simulink model "PV"  (R2024a)
settings: Solver=VariableStepAuto  StartTime=0.0  StopTime=0.5  RelTol=1e-3
libraries: ee_lib x48, nesl_utility x5, fl_lib x4, simulink x1, spspowerguiLib x1
settings Model: Creator=hp  LastModifiedBy=hp

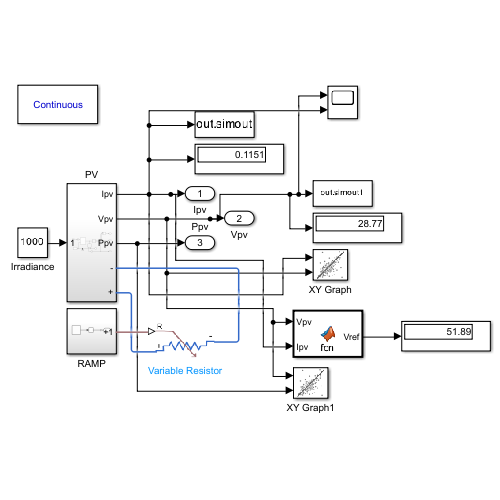
[thumbnail: Simulink's stored preview of the top-level diagram]
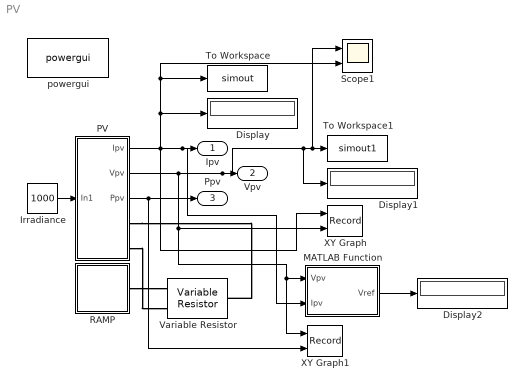
== system PV ==
  Display : Display
  Display1 : Display
  Display2 : Display
  Irradiance : Constant  Value=1000
  MATLAB Function : MATLAB Function  TreatAsAtomicUnit=on
  PV : Subsystem
  RAMP : Subsystem
  Scope1 : Scope  NumInputPorts=2
  To Workspace : ToWorkspace  VariableName=simout  SaveFormat=Timeseries  SampleTime=-1
  To Workspace1 : ToWorkspace  VariableName=simout1  SaveFormat=Timeseries  SampleTime=-1
  Variable Resistor : fl_lib/Electrical/Electrical Elements/Variable Resistor  Rmin=0 Ohm  thermalEnable=false  thermal_mass=1 J/K  i_specify=off  i_priority=None  i=0 A  i_nominal_specify=off  i_nominal_value=1  i_nominal_unit=A  v_specify=off  v_priority=None  v=0 V  v_nominal_specify=off  v_nominal_value=1  v_nominal_unit=V  T_specify=off  T_priority=None  T=300 K  T_nominal_specify=off  T_nominal_value=1  T_nominal_unit=K
  XY Graph : Record  FileSettingsInternal="{\"entries\":[{\"content\":{\"excelSettings\":{\"content\":{},\"type\":\"Streamout.ExcelSettings\"}},\"type\":\"Streamout.FileSettingStorage\",\"uuid\":\"\"}],\"packageUris\":[\"http:\\/\\/schema.mathworks.com\\/mf0\\/streamout_blocks\\/R2020a\"],\"version\":\"1.0\"}"  Layout=[1 1]  SignalsInternal="{\"entries\":[{\"content\":{\"signals\":[{\"content\":{\"blockPath\":[],\"dimensions\":[1],\"domain\":\"\",\"lineColor\":\"#a2142f\",\"plots\":[ 1 ],\"port\":1,\"signalID\":1,\"signalName\":\"PV:1\"},\"type\":\"RecordBlkView.Signal\",\"uuid\":\"\"},{\"content\":{\"blockPath\":[],\"dimensions\":[1],\"domain\":\"\",\"lineColor\":\"#139fff\",\"plots\":[ 1 ],\"port\":2,\"signalID\":2,\"signalName\":\"PV:2\"},\"type\":\"RecordBlkView.Signal\",\"uuid\":\"\"}]},\"type\":\"RecordBlkView.InputSignals\",\"uuid\":\"\"}],\"packageUris\":[\"http:\\/\\/schema.mathworks.com\\/mf0\\/streamout_blocks\\/R2020a\"],\"version\":\"1.0\"}"  VisualizationBindings="{\"xyplotplugin\":{\"info\":[{\"series\":[{\"bindingParametersList\":[{\"parameter\":\"X-Axis\",\"signalID\":1,\"signalName\":\"PV:1\"},{\"parameter\":\"Y-Axis\",\"signalID\":2,\"signalName\":\"PV:2\"}],\"seriesID\":0}],\"subplotID\":1}]}}"  CompatibilityTag=XY
  XY Graph1 : Record  FileSettingsInternal="{\"entries\":[{\"content\":{\"excelSettings\":{\"content\":{},\"type\":\"Streamout.ExcelSettings\"}},\"type\":\"Streamout.FileSettingStorage\",\"uuid\":\"\"}],\"packageUris\":[\"http:\\/\\/schema.mathworks.com\\/mf0\\/streamout_blocks\\/R2020a\"],\"version\":\"1.0\"}"  Layout=[1 1]  SignalsInternal="{\"entries\":[{\"content\":{\"signals\":[{\"content\":{\"blockPath\":[],\"dimensions\":[1],\"domain\":\"\",\"lineColor\":\"#a2142f\",\"plots\":[ 1 ],\"port\":1,\"signalID\":1,\"signalName\":\"Vpv\"},\"type\":\"RecordBlkView.Signal\",\"uuid\":\"\"},{\"content\":{\"blockPath\":[],\"dimensions\":[1],\"domain\":\"\",\"lineColor\":\"#139fff\",\"plots\":[ 1 ],\"port\":2,\"signalID\":2,\"signalName\":\"Ppv\"},\"type\":\"RecordBlkView.Signal\",\"uuid\":\"\"}]},\"type\":\"RecordBlkView.InputSignals\",\"uuid\":\"\"}],\"packageUris\":[\"http:\\/\\/schema.mathworks.com\\/mf0\\/streamout_blocks\\/R2020a\"],\"version\":\"1.0\"}"  VisualizationBindings="{\"xyplotplugin\":{\"info\":[{\"series\":[{\"bindingParametersList\":[{\"parameter\":\"X-Axis\",\"signalID\":1,\"signalName\":\"Vpv\"},{\"parameter\":\"Y-Axis\",\"signalID\":2,\"signalName\":\"Ppv\"}],\"seriesID\":0}],\"subplotID\":1}]}}"  CompatibilityTag=XY
  powergui : spspowerguiLib/powergui  Priority=1  SimulationMode=Continuous  SampleTime=50e-6  frequency=60  Iterations=50  frequencyindice=60  Pbase=100e6  ErrMax=1e-4  UnitsV=kV  UnitsW=MW  buscounter=0  FunctionMessages=off  echomessages=off  EnableUseOfTLC=off  CurrentSourceSwitches=off  DisableSnubberDevices=off  DisableRonSwitches=off  DisableVfSwitches=off  DisplayEquations=off  AutomaticDiscreteSolvers=off  SolverType=Tustin/Backward Euler (TBE)  Interpol=off  ExternalGateDelay=off  methode=off  Ts=100  x0status=blocks  SPID=on  SwTol=0  HookPort=off  NonlinearTolerance=1e-4  nMaxIteration=100  ContinueOnMaxIteration=off  RestoreLinks=warning  ResistiveCurrentMeasurement=off  Frange=[0:2:500]  Ylog=off  Xlog=on  ShowGrid=off  save=off  variable=ZData  structure=0  ZoomFFT=off  StartTime=0.0  cycles=1  DisplayStyle=1  fundamental=60  FreqAxis=off  MaxFrequency=1000  frequencyindicesteady=1  RmsSteady=1  display=off
  Ipv : Outport
  Vpv : Outport  Port=2
  Ppv : Outport  Port=3
  wires:
  Irradiance/1 -> PV/1(In1)
  PV/1(Ipv) -> XY Graph/1, Scope1/2, To Workspace/1, Display/1, MATLAB Function/2(Ipv), Ipv/1
  PV/3(Ppv) -> XY Graph1/2, Ppv/1
  PV/2(Vpv) -> XY Graph1/1, MATLAB Function/1(Vpv), XY Graph/2, Vpv/1, Scope1/1, To Workspace1/1, Display1/1
  MATLAB Function/1(Vref) -> Display2/1
  connections:
  PV/RConn2 -- Variable Resistor/LConn2
  PV/RConn1 -- Variable Resistor/RConn1
  RAMP/RConn1 -- Variable Resistor/LConn1

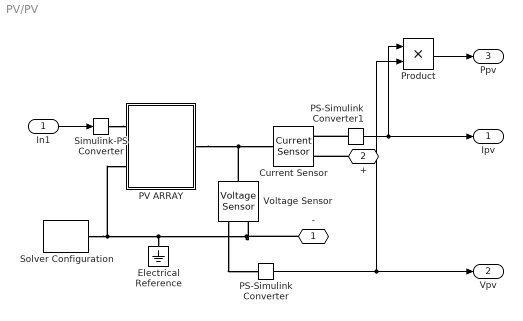
== system PV/PV ==
  In1 : Inport
  Current Sensor : fl_lib/Electrical/Electrical Sensors/Current Sensor
  Electrical Reference : fl_lib/Electrical/Electrical Elements/Electrical Reference
  PS-Simulink Converter : nesl_utility/PS-Simulink Converter  PhysicalDomain=network_engine_domain  SubClassName=ps_output  LeftPortType=input  RightPortType=output  PseudoPeriodic=off  Frequencies=[]  VectorFormat=inherit  Unit=inherit  AffineConversion=off
  PS-Simulink Converter1 : nesl_utility/PS-Simulink Converter  PhysicalDomain=network_engine_domain  SubClassName=ps_output  LeftPortType=input  RightPortType=output  PseudoPeriodic=off  Frequencies=[]  VectorFormat=inherit  Unit=inherit  AffineConversion=off
  PV ARRAY : Subsystem
  Product : Product
  Simulink-PS Converter : nesl_utility/Simulink-PS Converter  PhysicalDomain=network_engine_domain  SubClassName=ps_input  LeftPortType=input  RightPortType=output  PseudoPeriodic=off  Frequencies=[]  NoiseDistribution=none  NoiseParameters=[]  Unit=1  AffineConversion=off  FilteringAndDerivatives=provide  SimscapeFilterOrder=1  InputFilterTimeConstant=0.001  UdotUserProvided=0
  Solver Configuration : nesl_utility/Solver Configuration  PhysicalDomain=network_engine_domain  SubClassName=solver  LeftPortType=input  RightPortType=generic  Tones=[]  Harmonics=[]  SimulateNoise=off  Profile=off  UseLocalSampling=off  EnableSwitchedLinearOptims=on  FrequencyDomain=off  UseCCode=off  RelTol=0.001  AbsTol=0.001  MinStep=1e-09  ToWorkspace=off  RevertToSquareIcSolve=off  NumHomotopyIterations=100  PhasorMode=off  PhasorModeNumHarmonics=1  ConsistencySolver=NEWTON_XTOL_AFTER_FTOL  IndexReductionMethod=DerivativeReplacement  DoDC=off  ResidualTolerance=1e-09  ConsistencyTolSource=GLOBAL  ConsistencyAbsTol=0.001  ConsistencyRelTol=0.001  ConsistencyTolFactor=0.001  UseLocalSolver=off  LocalSolverChoice=NE_BACKWARD_EULER_ADVANCER  ResolveIndetEquations=on  FunctionEvalNumThread=1  LocalSolverSampleTime=0.001  DoFixedCost=off  MaxNonlinIter=3  MaxModeIter=2  ComputeImpulses=off  ImpulseIterations=2  LinearAlgebra=auto  LinearAlgebraNumThread=0  EquationFormulation=NE_TIME_EF  DelaysMemoryBudget=1024  AutomaticFiltering=on  FilteringTimeConstant=0.001  PartitionStorageMethod=AS_NEEDED  PartitionMemoryBudget=1024  PartitionMethod=ROBUST  MultibodyUseLocalSolver=off  MultibodyLocalSolverChoice=ODE1  MultibodyLocalSolverSampleTime=0.001
  Voltage Sensor : fl_lib/Electrical/Electrical Sensors/Voltage Sensor
  - : PMIOPort  Side=Right
  + : PMIOPort  Port=2  Side=Right
  Ipv : Outport
  Vpv : Outport  Port=2
  Ppv : Outport  Port=3
  wires:
  PS-Simulink Converter1/1 -> Ipv/1, Product/1
  PS-Simulink Converter/1 -> Vpv/1, Product/2
  Product/1 -> Ppv/1
  In1/1 -> Simulink-PS Converter/1
  connections:
  PS-Simulink Converter1/LConn1 -- Current Sensor/RConn1
  Simulink-PS Converter/RConn1 -- PV ARRAY/LConn1
  +/RConn1 -- Current Sensor/RConn2
  PV ARRAY/RConn1 -- Voltage Sensor/LConn1 -- Current Sensor/LConn1
  Solver Configuration/RConn1 -- -/RConn1 -- Voltage Sensor/RConn2 -- Electrical Reference/LConn1 -- PV ARRAY/LConn2
  Voltage Sensor/RConn1 -- PS-Simulink Converter/LConn1

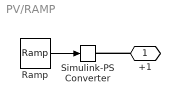
== system PV/RAMP ==
  Ramp : simulink/Sources/Ramp  slope=500  start=0  InitialOutput=0
  Simulink-PS Converter : nesl_utility/Simulink-PS Converter  PhysicalDomain=network_engine_domain  SubClassName=ps_input  LeftPortType=input  RightPortType=output  PseudoPeriodic=off  Frequencies=[]  NoiseDistribution=none  NoiseParameters=[]  Unit=1  AffineConversion=off  FilteringAndDerivatives=provide  SimscapeFilterOrder=1  InputFilterTimeConstant=0.001  UdotUserProvided=0
  +1 : PMIOPort  Side=Right
  wires:
  Ramp/1 -> Simulink-PS Converter/1
  connections:
  +1/RConn1 -- Simulink-PS Converter/RConn1

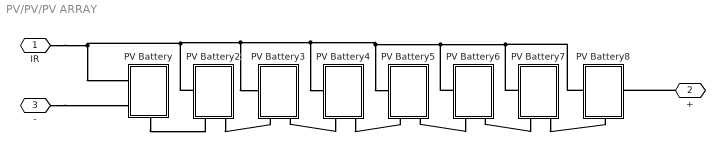
== system PV/PV/PV ARRAY ==
  PV Battery : Subsystem
      settings: PortSchema="{\"entries\":[{\"content\":{\"sides\":[{\"content\":{\"connectorIds\":[\"LConn1\",\"LConn2\"]},\"type\":\"ConnectorPlacement.EquallySpacedRectSide\",\"uuid\":\"343a5c80-c490-4c63-968f-4227f8b0bc69\"},{\"content\":{\"side\":\"RIGHT\"},\"type\":\"ConnectorPlacement.EquallySpacedRectSide\",\"uuid\":\"ee4aa178-7663-40d5-bcc3-f91d4c44b2a7\"},{\"content\":{\"side\":\"TOP\"},\"type\":\"ConnectorPlacement.EquallySpacedRectSide\",\"uuid\":\"a03aa1aa-4889-4cfe-9c8f-92adc9f70735\"},{\"content\":{\"connectorIds\":[\"RConn1\"],\"side\":\"BOTTOM\"},\"type\":\"ConnectorPlacement.EquallySpacedRectSide\",\"uuid\":\"9e292261-11b5-43da-a6bc-bd19848d4a2b\"}]},\"type\":\"ConnectorPlacement.EquallySpacedConnector\",\"uuid\":\"be6337a3-66bb-48d6-bc68-5a7e39297b74\"}],\"packageUris\":[\"http://schema.mathworks.com/mf0/Connector/R2020b\"],\"version\":\"1.0\"}"
  PV Battery2 : Subsystem
      settings: PortSchema="{\"entries\":[{\"content\":{\"sides\":[{\"content\":{\"connectorIds\":[\"LConn1\"]},\"type\":\"ConnectorPlacement.EquallySpacedRectSide\",\"uuid\":\"343a5c80-c490-4c63-968f-4227f8b0bc69\"},{\"content\":{\"side\":\"RIGHT\"},\"type\":\"ConnectorPlacement.EquallySpacedRectSide\",\"uuid\":\"ee4aa178-7663-40d5-bcc3-f91d4c44b2a7\"},{\"content\":{\"side\":\"TOP\"},\"type\":\"ConnectorPlacement.EquallySpacedRectSide\",\"uuid\":\"a03aa1aa-4889-4cfe-9c8f-92adc9f70735\"},{\"content\":{\"connectorIds\":[\"RConn1\",\"RConn2\"],\"side\":\"BOTTOM\"},\"type\":\"ConnectorPlacement.EquallySpacedRectSide\",\"uuid\":\"35521834-7b12-4f19-8790-069a58e4d08c\"}]},\"type\":\"ConnectorPlacement.EquallySpacedConnector\",\"uuid\":\"be6337a3-66bb-48d6-bc68-5a7e39297b74\"}],\"packageUris\":[\"http://schema.mathworks.com/mf0/Connector/R2020b\"],\"version\":\"1.0\"}"
  PV Battery3 : Subsystem
      settings: PortSchema="{\"entries\":[{\"content\":{\"sides\":[{\"content\":{\"connectorIds\":[\"LConn1\"]},\"type\":\"ConnectorPlacement.EquallySpacedRectSide\",\"uuid\":\"343a5c80-c490-4c63-968f-4227f8b0bc69\"},{\"content\":{\"side\":\"RIGHT\"},\"type\":\"ConnectorPlacement.EquallySpacedRectSide\",\"uuid\":\"ee4aa178-7663-40d5-bcc3-f91d4c44b2a7\"},{\"content\":{\"side\":\"TOP\"},\"type\":\"ConnectorPlacement.EquallySpacedRectSide\",\"uuid\":\"a03aa1aa-4889-4cfe-9c8f-92adc9f70735\"},{\"content\":{\"connectorIds\":[\"RConn1\",\"RConn2\"],\"side\":\"BOTTOM\"},\"type\":\"ConnectorPlacement.EquallySpacedRectSide\",\"uuid\":\"3f39185d-c5ea-40de-b77a-797dfb5d777b\"}]},\"type\":\"ConnectorPlacement.EquallySpacedConnector\",\"uuid\":\"be6337a3-66bb-48d6-bc68-5a7e39297b74\"}],\"packageUris\":[\"http://schema.mathworks.com/mf0/Connector/R2020b\"],\"version\":\"1.0\"}"
  PV Battery4 : Subsystem
      settings: PortSchema="{\"entries\":[{\"content\":{\"sides\":[{\"content\":{\"connectorIds\":[\"LConn1\"]},\"type\":\"ConnectorPlacement.EquallySpacedRectSide\",\"uuid\":\"343a5c80-c490-4c63-968f-4227f8b0bc69\"},{\"content\":{\"side\":\"RIGHT\"},\"type\":\"ConnectorPlacement.EquallySpacedRectSide\",\"uuid\":\"ee4aa178-7663-40d5-bcc3-f91d4c44b2a7\"},{\"content\":{\"side\":\"TOP\"},\"type\":\"ConnectorPlacement.EquallySpacedRectSide\",\"uuid\":\"a03aa1aa-4889-4cfe-9c8f-92adc9f70735\"},{\"content\":{\"connectorIds\":[\"RConn1\",\"RConn2\"],\"side\":\"BOTTOM\"},\"type\":\"ConnectorPlacement.EquallySpacedRectSide\",\"uuid\":\"6de3b158-1ff0-4b44-8b1b-28764e596168\"}]},\"type\":\"ConnectorPlacement.EquallySpacedConnector\",\"uuid\":\"be6337a3-66bb-48d6-bc68-5a7e39297b74\"}],\"packageUris\":[\"http://schema.mathworks.com/mf0/Connector/R2020b\"],\"version\":\"1.0\"}"
  PV Battery5 : Subsystem
      settings: PortSchema="{\"entries\":[{\"content\":{\"sides\":[{\"content\":{\"connectorIds\":[\"LConn1\"]},\"type\":\"ConnectorPlacement.EquallySpacedRectSide\",\"uuid\":\"343a5c80-c490-4c63-968f-4227f8b0bc69\"},{\"content\":{\"side\":\"RIGHT\"},\"type\":\"ConnectorPlacement.EquallySpacedRectSide\",\"uuid\":\"ee4aa178-7663-40d5-bcc3-f91d4c44b2a7\"},{\"content\":{\"side\":\"TOP\"},\"type\":\"ConnectorPlacement.EquallySpacedRectSide\",\"uuid\":\"a03aa1aa-4889-4cfe-9c8f-92adc9f70735\"},{\"content\":{\"connectorIds\":[\"RConn1\",\"RConn2\"],\"side\":\"BOTTOM\"},\"type\":\"ConnectorPlacement.EquallySpacedRectSide\",\"uuid\":\"8bb7a49a-a7b0-4dc7-aec8-a84a106abde2\"}]},\"type\":\"ConnectorPlacement.EquallySpacedConnector\",\"uuid\":\"be6337a3-66bb-48d6-bc68-5a7e39297b74\"}],\"packageUris\":[\"http://schema.mathworks.com/mf0/Connector/R2020b\"],\"version\":\"1.0\"}"
  PV Battery6 : Subsystem
      settings: PortSchema="{\"entries\":[{\"content\":{\"sides\":[{\"content\":{\"connectorIds\":[\"LConn1\"]},\"type\":\"ConnectorPlacement.EquallySpacedRectSide\",\"uuid\":\"343a5c80-c490-4c63-968f-4227f8b0bc69\"},{\"content\":{\"side\":\"RIGHT\"},\"type\":\"ConnectorPlacement.EquallySpacedRectSide\",\"uuid\":\"ee4aa178-7663-40d5-bcc3-f91d4c44b2a7\"},{\"content\":{\"side\":\"TOP\"},\"type\":\"ConnectorPlacement.EquallySpacedRectSide\",\"uuid\":\"a03aa1aa-4889-4cfe-9c8f-92adc9f70735\"},{\"content\":{\"connectorIds\":[\"RConn1\",\"RConn2\"],\"side\":\"BOTTOM\"},\"type\":\"ConnectorPlacement.EquallySpacedRectSide\",\"uuid\":\"8bb7a49a-a7b0-4dc7-aec8-a84a106abde2\"}]},\"type\":\"ConnectorPlacement.EquallySpacedConnector\",\"uuid\":\"be6337a3-66bb-48d6-bc68-5a7e39297b74\"}],\"packageUris\":[\"http://schema.mathworks.com/mf0/Connector/R2020b\"],\"version\":\"1.0\"}"
  PV Battery7 : Subsystem
      settings: PortSchema="{\"entries\":[{\"content\":{\"sides\":[{\"content\":{\"connectorIds\":[\"LConn1\"]},\"type\":\"ConnectorPlacement.EquallySpacedRectSide\",\"uuid\":\"343a5c80-c490-4c63-968f-4227f8b0bc69\"},{\"content\":{\"side\":\"RIGHT\"},\"type\":\"ConnectorPlacement.EquallySpacedRectSide\",\"uuid\":\"ee4aa178-7663-40d5-bcc3-f91d4c44b2a7\"},{\"content\":{\"side\":\"TOP\"},\"type\":\"ConnectorPlacement.EquallySpacedRectSide\",\"uuid\":\"a03aa1aa-4889-4cfe-9c8f-92adc9f70735\"},{\"content\":{\"connectorIds\":[\"RConn1\",\"RConn2\"],\"side\":\"BOTTOM\"},\"type\":\"ConnectorPlacement.EquallySpacedRectSide\",\"uuid\":\"8bb7a49a-a7b0-4dc7-aec8-a84a106abde2\"}]},\"type\":\"ConnectorPlacement.EquallySpacedConnector\",\"uuid\":\"be6337a3-66bb-48d6-bc68-5a7e39297b74\"}],\"packageUris\":[\"http://schema.mathworks.com/mf0/Connector/R2020b\"],\"version\":\"1.0\"}"
  PV Battery8 : Subsystem
      settings: PortSchema="{\"entries\":[{\"content\":{\"sides\":[{\"content\":{\"connectorIds\":[\"LConn1\"]},\"type\":\"ConnectorPlacement.EquallySpacedRectSide\",\"uuid\":\"343a5c80-c490-4c63-968f-4227f8b0bc69\"},{\"content\":{\"connectorIds\":[\"RConn1\"],\"side\":\"RIGHT\"},\"type\":\"ConnectorPlacement.EquallySpacedRectSide\",\"uuid\":\"ee4aa178-7663-40d5-bcc3-f91d4c44b2a7\"},{\"content\":{\"side\":\"TOP\"},\"type\":\"ConnectorPlacement.EquallySpacedRectSide\",\"uuid\":\"a03aa1aa-4889-4cfe-9c8f-92adc9f70735\"},{\"content\":{\"connectorIds\":[\"RConn2\"],\"side\":\"BOTTOM\"},\"type\":\"ConnectorPlacement.EquallySpacedRectSide\",\"uuid\":\"8bb7a49a-a7b0-4dc7-aec8-a84a106abde2\"}]},\"type\":\"ConnectorPlacement.EquallySpacedConnector\",\"uuid\":\"be6337a3-66bb-48d6-bc68-5a7e39297b74\"}],\"packageUris\":[\"http://schema.mathworks.com/mf0/Connector/R2020b\"],\"version\":\"1.0\"}"
  IR : PMIOPort  Side=Left
  + : PMIOPort  Port=2  Side=Right
  - : PMIOPort  Port=3  Side=Left
  connections:
  PV Battery2/LConn1 -- IR/RConn1 -- PV Battery/LConn1 -- PV Battery6/LConn1 -- PV Battery8/LConn1 -- PV Battery7/LConn1 -- PV Battery5/LConn1 -- PV Battery4/LConn1 -- PV Battery3/LConn1
  PV Battery/RConn1 -- PV Battery2/RConn1
  -/RConn1 -- PV Battery/LConn2
  PV Battery7/RConn2 -- PV Battery8/RConn2
  PV Battery2/RConn2 -- PV Battery3/RConn1
  PV Battery6/RConn1 -- PV Battery5/RConn2
  PV Battery4/RConn1 -- PV Battery3/RConn2
  PV Battery4/RConn2 -- PV Battery5/RConn1
  +/RConn1 -- PV Battery8/RConn1
  PV Battery7/RConn1 -- PV Battery6/RConn2

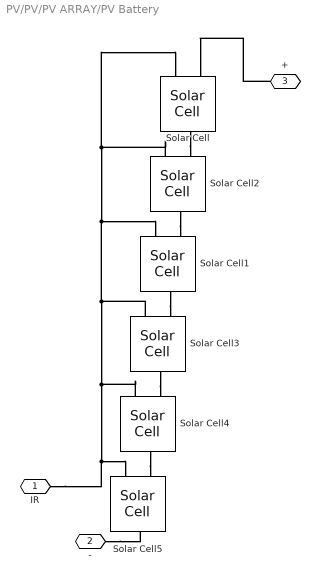
== system PV/PV/PV ARRAY/PV Battery ==
  Solar Cell{,1..5} (6 alike) : ee_lib/Sources/Solar Cell  prm=1  Isc=7.34 A  Voc=0.6 V  Is=1e-6 A  Is2=0 A  Iph=7.34 A  Ir0=1000 W/m^2  ec=1.5  N2=2  Rs=0 Ohm  Rp=inf Ohm  N_series=1  N_parallel=1  TIPH1=0 1/K  EG=1.11 eV  TXIS1=3  TXIS2=3  TRS1=0  TRP1=0  Tmeas=25 degC  TFIXED=25 degC  thermal_mass=100 J/K  initial_temperature=25 degC
  IR : PMIOPort  Side=Left
  - : PMIOPort  Port=2  Side=Left
  + : PMIOPort  Port=3  Side=Right
  connections:
  Solar Cell2/LConn1 -- Solar Cell/LConn1 -- Solar Cell3/LConn1 -- Solar Cell4/LConn1 -- IR/RConn1 -- Solar Cell5/LConn1 -- Solar Cell1/LConn1
  Solar Cell/RConn1 -- Solar Cell2/LConn2
  Solar Cell4/RConn1 -- Solar Cell5/LConn2
  +/RConn1 -- Solar Cell/LConn2
  Solar Cell1/RConn1 -- Solar Cell3/LConn2
  Solar Cell3/RConn1 -- Solar Cell4/LConn2
  -/RConn1 -- Solar Cell5/RConn1
  Solar Cell2/RConn1 -- Solar Cell1/LConn2

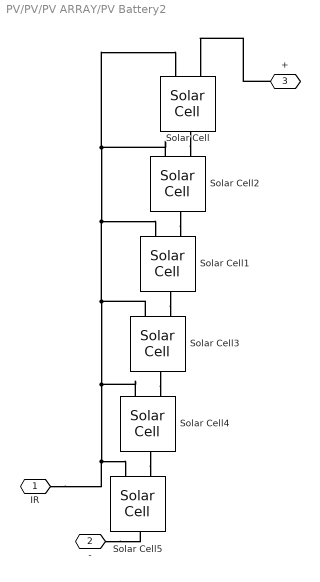
== system PV/PV/PV ARRAY/PV Battery2 ==
  Solar Cell{,1..5} (6 alike) : ee_lib/Sources/Solar Cell  prm=1  Isc=7.34 A  Voc=0.6 V  Is=1e-6 A  Is2=0 A  Iph=7.34 A  Ir0=1000 W/m^2  ec=1.5  N2=2  Rs=0 Ohm  Rp=inf Ohm  N_series=1  N_parallel=1  TIPH1=0 1/K  EG=1.11 eV  TXIS1=3  TXIS2=3  TRS1=0  TRP1=0  Tmeas=25 degC  TFIXED=25 degC  thermal_mass=100 J/K  initial_temperature=25 degC
  IR : PMIOPort  Side=Left
  - : PMIOPort  Port=2  Side=Right
  + : PMIOPort  Port=3  Side=Right
  connections:
  Solar Cell4/LConn1 -- Solar Cell3/LConn1 -- Solar Cell2/LConn1 -- Solar Cell/LConn1 -- Solar Cell1/LConn1 -- Solar Cell5/LConn1 -- IR/RConn1
  Solar Cell/RConn1 -- Solar Cell2/LConn2
  Solar Cell4/RConn1 -- Solar Cell5/LConn2
  +/RConn1 -- Solar Cell/LConn2
  Solar Cell1/RConn1 -- Solar Cell3/LConn2
  Solar Cell3/RConn1 -- Solar Cell4/LConn2
  -/RConn1 -- Solar Cell5/RConn1
  Solar Cell2/RConn1 -- Solar Cell1/LConn2

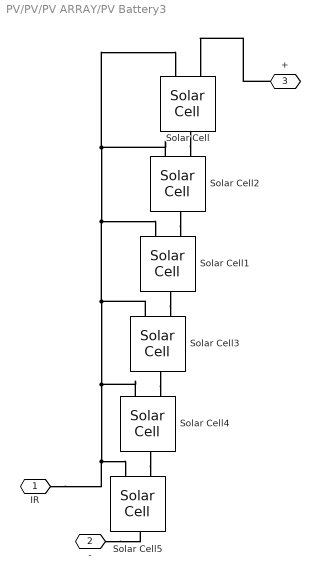
== system PV/PV/PV ARRAY/PV Battery3 ==
  Solar Cell{,1..5} (6 alike) : ee_lib/Sources/Solar Cell  prm=1  Isc=7.34 A  Voc=0.6 V  Is=1e-6 A  Is2=0 A  Iph=7.34 A  Ir0=1000 W/m^2  ec=1.5  N2=2  Rs=0 Ohm  Rp=inf Ohm  N_series=1  N_parallel=1  TIPH1=0 1/K  EG=1.11 eV  TXIS1=3  TXIS2=3  TRS1=0  TRP1=0  Tmeas=25 degC  TFIXED=25 degC  thermal_mass=100 J/K  initial_temperature=25 degC
  IR : PMIOPort  Side=Left
  - : PMIOPort  Port=2  Side=Right
  + : PMIOPort  Port=3  Side=Right
  connections:
  Solar Cell4/LConn1 -- Solar Cell3/LConn1 -- Solar Cell2/LConn1 -- Solar Cell/LConn1 -- Solar Cell1/LConn1 -- Solar Cell5/LConn1 -- IR/RConn1
  Solar Cell/RConn1 -- Solar Cell2/LConn2
  Solar Cell4/RConn1 -- Solar Cell5/LConn2
  +/RConn1 -- Solar Cell/LConn2
  Solar Cell1/RConn1 -- Solar Cell3/LConn2
  Solar Cell3/RConn1 -- Solar Cell4/LConn2
  -/RConn1 -- Solar Cell5/RConn1
  Solar Cell2/RConn1 -- Solar Cell1/LConn2

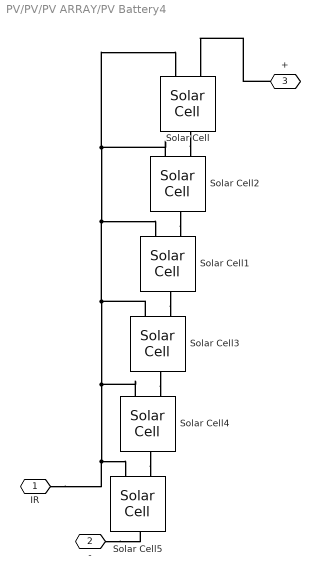
== system PV/PV/PV ARRAY/PV Battery4 ==
  Solar Cell{,1..5} (6 alike) : ee_lib/Sources/Solar Cell  prm=1  Isc=7.34 A  Voc=0.6 V  Is=1e-6 A  Is2=0 A  Iph=7.34 A  Ir0=1000 W/m^2  ec=1.5  N2=2  Rs=0 Ohm  Rp=inf Ohm  N_series=1  N_parallel=1  TIPH1=0 1/K  EG=1.11 eV  TXIS1=3  TXIS2=3  TRS1=0  TRP1=0  Tmeas=25 degC  TFIXED=25 degC  thermal_mass=100 J/K  initial_temperature=25 degC
  IR : PMIOPort  Side=Left
  - : PMIOPort  Port=2  Side=Right
  + : PMIOPort  Port=3  Side=Right
  connections:
  Solar Cell4/LConn1 -- Solar Cell3/LConn1 -- Solar Cell2/LConn1 -- Solar Cell/LConn1 -- Solar Cell1/LConn1 -- Solar Cell5/LConn1 -- IR/RConn1
  Solar Cell/RConn1 -- Solar Cell2/LConn2
  Solar Cell4/RConn1 -- Solar Cell5/LConn2
  +/RConn1 -- Solar Cell/LConn2
  Solar Cell1/RConn1 -- Solar Cell3/LConn2
  Solar Cell3/RConn1 -- Solar Cell4/LConn2
  -/RConn1 -- Solar Cell5/RConn1
  Solar Cell2/RConn1 -- Solar Cell1/LConn2

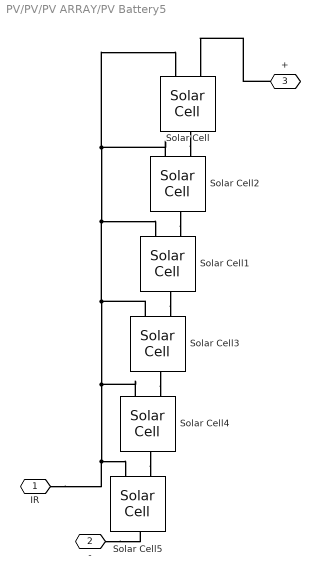
== system PV/PV/PV ARRAY/PV Battery5 ==
  Solar Cell{,1..5} (6 alike) : ee_lib/Sources/Solar Cell  prm=1  Isc=7.34 A  Voc=0.6 V  Is=1e-6 A  Is2=0 A  Iph=7.34 A  Ir0=1000 W/m^2  ec=1.5  N2=2  Rs=0 Ohm  Rp=inf Ohm  N_series=1  N_parallel=1  TIPH1=0 1/K  EG=1.11 eV  TXIS1=3  TXIS2=3  TRS1=0  TRP1=0  Tmeas=25 degC  TFIXED=25 degC  thermal_mass=100 J/K  initial_temperature=25 degC
  IR : PMIOPort  Side=Left
  - : PMIOPort  Port=2  Side=Right
  + : PMIOPort  Port=3  Side=Right
  connections:
  Solar Cell4/LConn1 -- Solar Cell3/LConn1 -- Solar Cell2/LConn1 -- Solar Cell/LConn1 -- Solar Cell1/LConn1 -- Solar Cell5/LConn1 -- IR/RConn1
  Solar Cell/RConn1 -- Solar Cell2/LConn2
  Solar Cell4/RConn1 -- Solar Cell5/LConn2
  +/RConn1 -- Solar Cell/LConn2
  Solar Cell1/RConn1 -- Solar Cell3/LConn2
  Solar Cell3/RConn1 -- Solar Cell4/LConn2
  -/RConn1 -- Solar Cell5/RConn1
  Solar Cell2/RConn1 -- Solar Cell1/LConn2

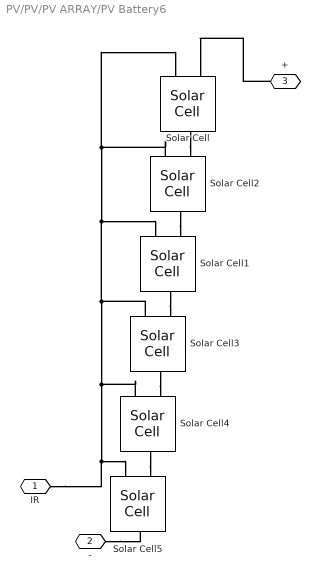
== system PV/PV/PV ARRAY/PV Battery6 ==
  Solar Cell{,1..5} (6 alike) : ee_lib/Sources/Solar Cell  prm=1  Isc=7.34 A  Voc=0.6 V  Is=1e-6 A  Is2=0 A  Iph=7.34 A  Ir0=1000 W/m^2  ec=1.5  N2=2  Rs=0 Ohm  Rp=inf Ohm  N_series=1  N_parallel=1  TIPH1=0 1/K  EG=1.11 eV  TXIS1=3  TXIS2=3  TRS1=0  TRP1=0  Tmeas=25 degC  TFIXED=25 degC  thermal_mass=100 J/K  initial_temperature=25 degC
  IR : PMIOPort  Side=Left
  - : PMIOPort  Port=2  Side=Right
  + : PMIOPort  Port=3  Side=Right
  connections:
  Solar Cell4/LConn1 -- Solar Cell3/LConn1 -- Solar Cell2/LConn1 -- Solar Cell/LConn1 -- Solar Cell1/LConn1 -- Solar Cell5/LConn1 -- IR/RConn1
  Solar Cell/RConn1 -- Solar Cell2/LConn2
  Solar Cell4/RConn1 -- Solar Cell5/LConn2
  +/RConn1 -- Solar Cell/LConn2
  Solar Cell1/RConn1 -- Solar Cell3/LConn2
  Solar Cell3/RConn1 -- Solar Cell4/LConn2
  -/RConn1 -- Solar Cell5/RConn1
  Solar Cell2/RConn1 -- Solar Cell1/LConn2

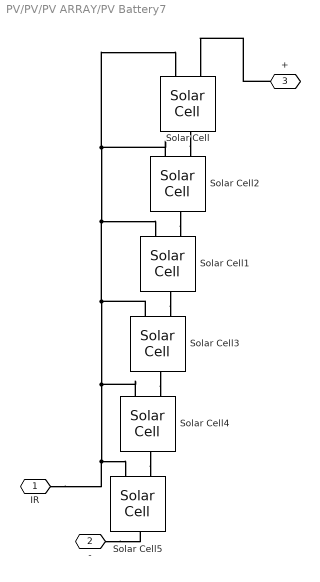
== system PV/PV/PV ARRAY/PV Battery7 ==
  Solar Cell{,1..5} (6 alike) : ee_lib/Sources/Solar Cell  prm=1  Isc=7.34 A  Voc=0.6 V  Is=1e-6 A  Is2=0 A  Iph=7.34 A  Ir0=1000 W/m^2  ec=1.5  N2=2  Rs=0 Ohm  Rp=inf Ohm  N_series=1  N_parallel=1  TIPH1=0 1/K  EG=1.11 eV  TXIS1=3  TXIS2=3  TRS1=0  TRP1=0  Tmeas=25 degC  TFIXED=25 degC  thermal_mass=100 J/K  initial_temperature=25 degC
  IR : PMIOPort  Side=Left
  - : PMIOPort  Port=2  Side=Right
  + : PMIOPort  Port=3  Side=Right
  connections:
  Solar Cell4/LConn1 -- Solar Cell3/LConn1 -- Solar Cell2/LConn1 -- Solar Cell/LConn1 -- Solar Cell1/LConn1 -- Solar Cell5/LConn1 -- IR/RConn1
  Solar Cell/RConn1 -- Solar Cell2/LConn2
  Solar Cell4/RConn1 -- Solar Cell5/LConn2
  +/RConn1 -- Solar Cell/LConn2
  Solar Cell1/RConn1 -- Solar Cell3/LConn2
  Solar Cell3/RConn1 -- Solar Cell4/LConn2
  -/RConn1 -- Solar Cell5/RConn1
  Solar Cell2/RConn1 -- Solar Cell1/LConn2

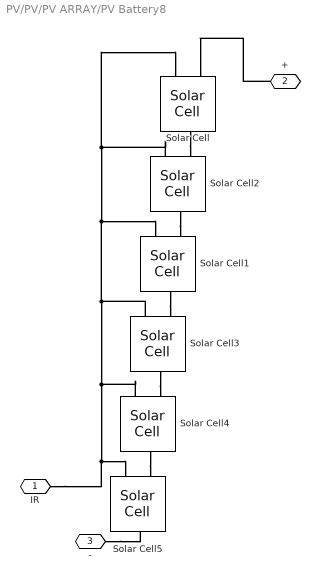
== system PV/PV/PV ARRAY/PV Battery8 ==
  Solar Cell{,1..5} (6 alike) : ee_lib/Sources/Solar Cell  prm=1  Isc=7.34 A  Voc=0.6 V  Is=1e-6 A  Is2=0 A  Iph=7.34 A  Ir0=1000 W/m^2  ec=1.5  N2=2  Rs=0 Ohm  Rp=inf Ohm  N_series=1  N_parallel=1  TIPH1=0 1/K  EG=1.11 eV  TXIS1=3  TXIS2=3  TRS1=0  TRP1=0  Tmeas=25 degC  TFIXED=25 degC  thermal_mass=100 J/K  initial_temperature=25 degC
  IR : PMIOPort  Side=Left
  + : PMIOPort  Port=2  Side=Right
  - : PMIOPort  Port=3  Side=Right
  connections:
  Solar Cell4/LConn1 -- Solar Cell3/LConn1 -- Solar Cell2/LConn1 -- Solar Cell/LConn1 -- Solar Cell1/LConn1 -- Solar Cell5/LConn1 -- IR/RConn1
  Solar Cell/RConn1 -- Solar Cell2/LConn2
  Solar Cell4/RConn1 -- Solar Cell5/LConn2
  +/RConn1 -- Solar Cell/LConn2
  Solar Cell1/RConn1 -- Solar Cell3/LConn2
  Solar Cell3/RConn1 -- Solar Cell4/LConn2
  -/RConn1 -- Solar Cell5/RConn1
  Solar Cell2/RConn1 -- Solar Cell1/LConn2

== matlab function PV/MATLAB Function ==
  data: Vpv input; Vref output; Ipv input
function Vref=fcn(Vpv,Ipv)
V=52;
I=0.001;
P=V*I;
c=0.11;
Pnew=Vpv*Ipv;
if (Pnew>P)
    if(Vpv>V)
        Vpv=V+c;
    else
        Vpv=V-c;
    end
else
    if(Vpv<V)
        Vpv=V+c;
    else
        Vpv=V-c;
    end
end
V=Vpv;
I=Ipv;
P=Pnew;
Vref=Vpv;
